simulink model "dyros_tocabi_0714"  (R2023a)
settings: Solver=VariableStepAuto  StartTime=0.0  StopTime=1.7995  RelTol=1e-3
undefined symbols (not defined in the file or in its folder): X, Y, Z
libraries: sm_lib x342, nesl_utility x36
(part 1 of 8)
settings Model: Creator=lhg08  LastModifiedBy=lhg08

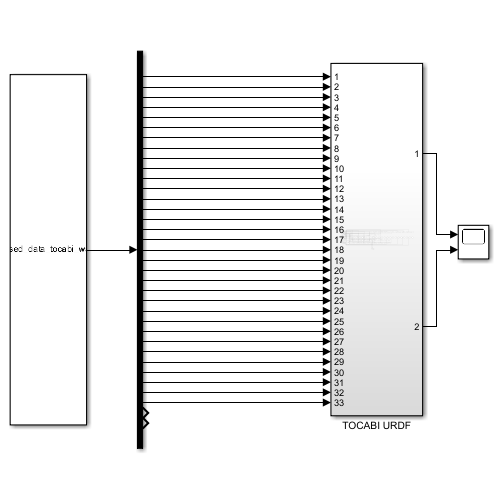
[thumbnail: Simulink's stored preview of the top-level diagram]
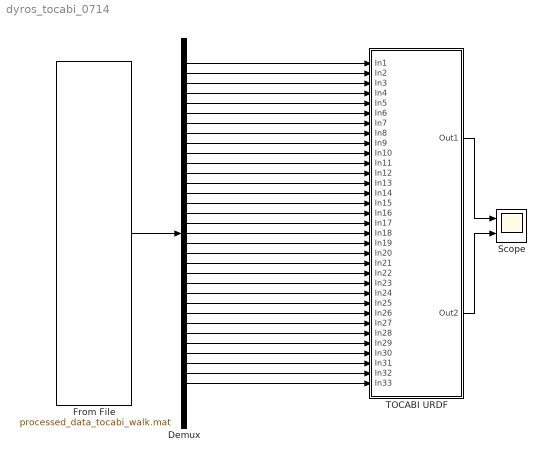
== system dyros_tocabi_0714 ==
  Demux : Demux  Outputs=35
  From File : FromFile  FileName=processed_data_tocabi_walk.mat  OutDataTypeStr=double  SampleTime=0
  Scope : Scope  NumInputPorts=2
  TOCABI URDF : Subsystem
  wires:
  Demux/1 -> TOCABI URDF/1(In1)
  Demux/33 -> TOCABI URDF/33(In33)
  Demux/32 -> TOCABI URDF/32(In32)
  Demux/30 -> TOCABI URDF/30(In30)
  Demux/31 -> TOCABI URDF/31(In31)
  Demux/2 -> TOCABI URDF/2(In2)
  Demux/4 -> TOCABI URDF/4(In4)
  Demux/3 -> TOCABI URDF/3(In3)
  Demux/5 -> TOCABI URDF/5(In5)
  Demux/6 -> TOCABI URDF/6(In6)
  Demux/7 -> TOCABI URDF/7(In7)
  Demux/8 -> TOCABI URDF/8(In8)
  Demux/9 -> TOCABI URDF/9(In9)
  Demux/10 -> TOCABI URDF/10(In10)
  Demux/12 -> TOCABI URDF/12(In12)
  Demux/11 -> TOCABI URDF/11(In11)
  Demux/13 -> TOCABI URDF/13(In13)
  Demux/14 -> TOCABI URDF/14(In14)
  Demux/15 -> TOCABI URDF/15(In15)
  Demux/16 -> TOCABI URDF/16(In16)
  Demux/17 -> TOCABI URDF/17(In17)
  Demux/18 -> TOCABI URDF/18(In18)
  Demux/19 -> TOCABI URDF/19(In19)
  Demux/20 -> TOCABI URDF/20(In20)
  Demux/21 -> TOCABI URDF/21(In21)
  Demux/22 -> TOCABI URDF/22(In22)
  Demux/23 -> TOCABI URDF/23(In23)
  Demux/24 -> TOCABI URDF/24(In24)
  Demux/25 -> TOCABI URDF/25(In25)
  Demux/26 -> TOCABI URDF/26(In26)
  Demux/27 -> TOCABI URDF/27(In27)
  Demux/28 -> TOCABI URDF/28(In28)
  Demux/29 -> TOCABI URDF/29(In29)
  From File/1 -> Demux/1
  TOCABI URDF/1(Out1) -> Scope/1
  TOCABI URDF/2(Out2) -> Scope/2
